simulink library "VISMODAL_MASTER"  (Simulink 8.6)
settings: Solver=VariableStepAuto  StartTime=0.0  StopTime=10.0  RelTol=1e-3
libraries: VIS_LIB x140, cdsFilt x34, cdsMuxMatrix x6, VISMODAL_MASTER x1
(part 2 of 5)

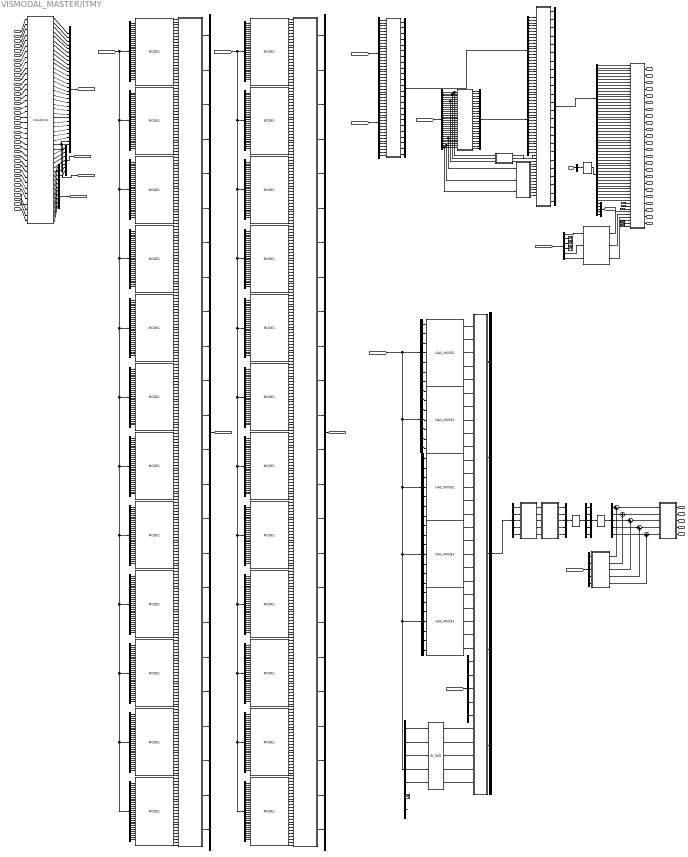
== system VISMODAL_MASTER/ITMY ==
  MCPS_V1 : Inport
  MCPS_V2 : Inport  Port=2
  MCPS_V3 : Inport  Port=3
  MCPS_H1 : Inport  Port=4
  MCPS_H2 : Inport  Port=5
  MCPS_H3 : Inport  Port=6
  IMPS_V1 : Inport  Port=7
  IMPS_V2 : Inport  Port=8
  IMPS_V3 : Inport  Port=9
  IMPS_H1 : Inport  Port=10
  IMPS_H2 : Inport  Port=11
  IMPS_H3 : Inport  Port=12
  TILT_SEG1 : Inport  Port=13
  TILT_SEG2 : Inport  Port=14
  TILT_SEG3 : Inport  Port=15
  TILT_SEG4 : Inport  Port=16
  LEN_SEG1 : Inport  Port=17
  LEN_SEG2 : Inport  Port=18
  LEN_SEG3 : Inport  Port=19
  LEN_SEG4 : Inport  Port=20
  BFLVDT_V1 : Inport  Port=21
  BFLVDT_V2 : Inport  Port=22
  BFLVDT_V3 : Inport  Port=23
  BFLVDT_H1 : Inport  Port=24
  BFLVDT_H2 : Inport  Port=25
  BFLVDT_H3 : Inport  Port=26
  IPLVDT_H1 : Inport  Port=27
  IPLVDT_H2 : Inport  Port=28
  IPLVDT_H3 : Inport  Port=29
  MNSEG1 : Inport  Port=30
  MNSEG2 : Inport  Port=31
  MNSEG3 : Inport  Port=32
  MNSEG4 : Inport  Port=33
  F0 : Inport  Port=34
  F1 : Inport  Port=35
  F2 : Inport  Port=36
  F3 : Inport  Port=37
  BF : Inport  Port=38
  QUAEXC : Inport  Port=39
  AI_GAS : Subsystem
  COILOUT_GAS : Subsystem
  DAMP : Subsystem
  DAMP_GAS : VISMODAL_MASTER/ITMY/AI_GAS
  DIAG : VIS_LIB/MODAL/inputproc
  DRIVEDECPL_GAS : cdsMuxMatrix/Subsystem  Tag=cdsMuxMatrix  Description=Any size matrix. Inputs and outputs must be connected using Mux and Demux parts.
      settings: AttributesFormatString=%<Tag>
  Demux{,2..24,27} (25 alike) : Demux  Outputs=30
  Demux{1,25..26,29,39} (5 alike) : Demux  Outputs=24
  Demux{28,30..33,41} (6 alike) : Demux  Outputs=7
  Demux{34..38} (5 alike) : Demux  Outputs=5
  Demux40 : Demux  Outputs=29
  Demux42 : Demux  Outputs=6
  EUL2COIL_GAS : cdsMuxMatrix/Subsystem  Tag=cdsMuxMatrix  Description=Any size matrix. Inputs and outputs must be connected using Mux and Demux parts.
      settings: AttributesFormatString=%<Tag>
  GASDC : Subsystem
  GAS_MODE{1..5} (5 alike) : VIS_LIB/MODAL/GAS_MODE1
  Ground{8..9,11,13,15,18} (6 alike) : Ground
  IPDC : Subsystem
  MNOL_SERVO_MN : Subsystem
  MODE{1..24} (24 alike) : VIS_LIB/MODAL/MODE1
  Mux : Mux  Inputs=30
  Mux{1..2,4..5,9} (5 alike) : Mux  Inputs=24
  Mux10 : Mux  Inputs=1
  Mux{6..8,11,13} (5 alike) : Mux  Inputs=5
  Mux12 : Mux  Inputs=6
  Mux3 : Mux  Inputs=7
  QUAEXC_SEL : cdsMuxMatrix/Subsystem  Tag=cdsMuxMatrix  Description=Any size matrix. Inputs and outputs must be connected using Mux and Demux parts.
      settings: AttributesFormatString=%<Tag>
  SUM_GAS : Subsystem
  Subsystem : Subsystem
  Sum{5..9} (5 alike) : Sum  Inputs=|++
  TMOL : Subsystem
  Terminator{,1..3} (4 alike) : Terminator
  sum : Subsystem
  sum1 : Subsystem
  sum10 : Subsystem
  sum2 : Subsystem
  sum3 : Subsystem
  IPLo : Outport
  IPTo : Outport  Port=2
  IPYo : Outport  Port=3
  BFLo : Outport  Port=4
  BFTo : Outport  Port=5
  BFVo : Outport  Port=6
  BFRo : Outport  Port=7
  BFPo : Outport  Port=8
  BFYo : Outport  Port=9
  MNLo : Outport  Port=10
  MNTo : Outport  Port=11
  MNVo : Outport  Port=12
  MNRo : Outport  Port=13
  MNPo : Outport  Port=14
  MNYo : Outport  Port=15
  IMLo : Outport  Port=16
  IMTo : Outport  Port=17
  IMVo : Outport  Port=18
  IMRo : Outport  Port=19
  IMPo : Outport  Port=20
  IMYo : Outport  Port=21
  TMLo : Outport  Port=22
  TMPo : Outport  Port=23
  TMYo : Outport  Port=24
  F0out : Outport  Port=25
  F1out : Outport  Port=26
  F2out : Outport  Port=27
  F3out : Outport  Port=28
  BFout : Outport  Port=29
  wires:
  Mux/1 -> [Signal]
  [Signal] -> Demux27/1
  DAMP/1(IPLo) -> Mux4/1
  DAMP/2(IPTo) -> Mux4/2
  DAMP/3(IPYo) -> Mux4/3
  DAMP/4(BFLo) -> Mux4/4
  DAMP/5(BFTo) -> Mux4/5
  DAMP/6(BFVo) -> Mux4/6
  DAMP/7(BFRo) -> Mux4/7
  DAMP/8(BFPo) -> Mux4/8
  DAMP/9(BFYo) -> Mux4/9
  DAMP/10(MNLo) -> Mux4/10
  DAMP/11(MNTo) -> Mux4/11
  DAMP/12(MNVo) -> Mux4/12
  DAMP/13(MNRo) -> Mux4/13
  DAMP/14(MNPo) -> Mux4/14
  DAMP/15(MNYo) -> Mux4/15
  DAMP/16(IMLo) -> Mux4/16
  DAMP/17(IMTo) -> Mux4/17
  DAMP/18(IMVo) -> Mux4/18
  DAMP/19(IMRo) -> Mux4/19
  DAMP/20(IMPo) -> Mux4/20
  DAMP/21(IMYo) -> Mux4/21
  DAMP/22(TMLo) -> Mux4/22
  DAMP/23(TMPo) -> Mux4/23
  DAMP/24(TMYo) -> Mux4/24
  Mux4/1 -> Demux29/1
  Demux29/1 -> sum10/25(IPL2)
  Demux29/2 -> sum10/26(IPT2)
  Demux29/3 -> sum10/27(IPY2)
  Demux29/4 -> sum10/28(BFL2)
  Demux29/5 -> sum10/29(BFT2)
  Demux29/6 -> sum10/30(BFV2)
  Demux29/7 -> sum10/31(BFR2)
  Demux29/8 -> sum10/32(BFP2)
  Demux29/9 -> sum10/33(BFY2)
  Demux29/10 -> sum10/34(MNL2)
  Demux29/11 -> sum10/35(MNT2)
  Demux29/12 -> sum10/36(MNV2)
  Demux29/13 -> sum10/37(MNR2)
  Demux29/14 -> sum10/38(MNP2)
  Demux29/15 -> sum10/39(MNY2)
  Demux29/16 -> sum10/40(IML2)
  Demux29/17 -> sum10/41(IMT2)
  Demux29/18 -> sum10/42(IMV2)
  Demux29/19 -> sum10/43(IMR2)
  Demux29/20 -> sum10/44(IMP2)
  Demux29/21 -> sum10/45(IMY2)
  Demux29/22 -> sum10/46(TML2)
  Demux29/23 -> sum10/47(TMP2)
  Demux29/24 -> sum10/48(TMY2)
  Demux27/1 -> IPDC/1(IPL), DAMP/1(IPL)
  Demux27/2 -> IPDC/2(IPT), DAMP/2(IPT)
  Demux27/3 -> DAMP/3(IPV)
  Demux27/4 -> DAMP/4(IPR)
  Demux27/5 -> DAMP/5(IPP)
  Demux27/6 -> IPDC/3(IPY), DAMP/6(IPY)
  Demux27/7 -> DAMP/7(BFL)
  Demux27/8 -> DAMP/8(BFT)
  Demux27/9 -> DAMP/9(BFV)
  Demux27/10 -> DAMP/10(BFR)
  Demux27/11 -> DAMP/11(BFP)
  Demux27/12 -> DAMP/12(BFY)
  Demux27/13 -> DAMP/13(MNL)
  Demux27/14 -> DAMP/14(MLT)
  Demux27/15 -> DAMP/15(MNV)
  Demux27/16 -> DAMP/16(MNR)
  Demux27/17 -> DAMP/17(MNP)
  Demux27/18 -> DAMP/18(MNY)
  Demux27/19 -> DAMP/19(IML)
  Demux27/20 -> DAMP/20(IMT)
  Demux27/21 -> DAMP/21(IMV)
  Demux27/22 -> DAMP/22(IMR)
  Demux27/23 -> DAMP/23(IMP)
  Demux27/24 -> DAMP/24(IMY)
  Demux27/26 -> DAMP/26(TMT)
  Demux27/27 -> DAMP/27(TMV)
  Demux27/28 -> DAMP/28(TMR)
  Demux27/29 -> TMOL/2(OLP), DAMP/29(TMP)
  Demux27/30 -> TMOL/3(OLY), DAMP/30(TMY)
  DIAG/1 -> Mux/1
  DIAG/2 -> Mux/2
  DIAG/3 -> Mux/3
  DIAG/4 -> Mux/4
  DIAG/5 -> Mux/5
  DIAG/6 -> Mux/6
  DIAG/7 -> Mux/7
  DIAG/8 -> Mux/8
  DIAG/9 -> Mux/9
  DIAG/10 -> Mux/10
  DIAG/11 -> Mux/11
  DIAG/12 -> Mux/12
  DIAG/13 -> Mux/13
  DIAG/14 -> Mux/14
  DIAG/15 -> Mux/15
  DIAG/16 -> Mux/16
  DIAG/17 -> Mux/17
  DIAG/18 -> Mux/18
  DIAG/19 -> Mux/19
  DIAG/20 -> Mux/20
  DIAG/21 -> Mux/21
  DIAG/22 -> Mux/22
  DIAG/23 -> Mux/23
  DIAG/24 -> Mux/24
  DIAG/25 -> Mux/25
  DIAG/26 -> Mux/26
  DIAG/27 -> Mux/27
  DIAG/28 -> Mux/28
  DIAG/29 -> Mux3/6, Mux/29
  DIAG/30 -> Mux3/7, Mux/30
  IPLVDT_H1/1 -> DIAG/1
  IPLVDT_H2/1 -> DIAG/2
  IPLVDT_H3/1 -> DIAG/3
  BFLVDT_V1/1 -> DIAG/4
  BFLVDT_V2/1 -> DIAG/5
  BFLVDT_V3/1 -> DIAG/6
  BFLVDT_H1/1 -> DIAG/7
  BFLVDT_H2/1 -> DIAG/8
  BFLVDT_H3/1 -> DIAG/9
  MCPS_V1/1 -> DIAG/10
  MCPS_V2/1 -> DIAG/11
  MCPS_V3/1 -> DIAG/12
  MCPS_H1/1 -> DIAG/13
  MCPS_H2/1 -> DIAG/14
  MCPS_H3/1 -> DIAG/15
  IMPS_V1/1 -> DIAG/16
  IMPS_V2/1 -> DIAG/17
  IMPS_V3/1 -> DIAG/18
  IMPS_H1/1 -> DIAG/19
  IMPS_H2/1 -> DIAG/20
  IMPS_H3/1 -> DIAG/21
  TILT_SEG1/1 -> DIAG/22
  TILT_SEG2/1 -> DIAG/23
  TILT_SEG3/1 -> DIAG/24
  TILT_SEG4/1 -> DIAG/25
  LEN_SEG1/1 -> DIAG/26
  LEN_SEG2/1 -> DIAG/27
  LEN_SEG3/1 -> DIAG/28
  LEN_SEG4/1 -> DIAG/29
  MNSEG2/1 -> DIAG/31
  MNSEG1/1 -> DIAG/30
  MNSEG3/1 -> DIAG/32
  MNSEG4/1 -> DIAG/33
  sum/1(IPL) -> Mux1/1
  sum/2(IPT) -> Mux1/2
  sum/3(IPY) -> Mux1/3
  sum/4(BFL) -> Mux1/4
  sum/5(BFT) -> Mux1/5
  sum/6(BFV) -> Mux1/6
  sum/7(BFR) -> Mux1/7
  sum/8(BFP) -> Mux1/8
  sum/9(BFY) -> Mux1/9
  sum/10(MNL) -> Mux1/10
  sum/11(MNT) -> Mux1/11
  sum/12(MNV) -> Mux1/12
  sum/13(MNR) -> Mux1/13
  sum/14(MNP) -> Mux1/14
  sum/15(MNY) -> Mux1/15
  sum/16(IML) -> Mux1/16
  sum/17(IMT) -> Mux1/17
  sum/18(IMV) -> Mux1/18
  sum/19(IMR) -> Mux1/19
  sum/20(IMP) -> Mux1/20
  sum/21(IMY) -> Mux1/21
  sum/22(TML) -> Mux1/22
  sum/23(TMP) -> Mux1/23
  sum/24(TMY) -> Mux1/24
  MODE1/1 -> sum/1(IPL1)
  MODE1/2 -> sum/2(IPT1)
  MODE1/3 -> sum/3(IPY1)
  MODE1/4 -> sum/4(BFL1)
  MODE1/5 -> sum/5(BFT1)
  MODE1/6 -> sum/6(BFV1)
  MODE1/7 -> sum/7(BFR1)
  MODE1/8 -> sum/8(BFP1)
  MODE1/9 -> sum/9(BFY1)
  MODE1/10 -> sum/10(MNL1)
  MODE1/11 -> sum/11(MNT1)
  MODE1/12 -> sum/12(MNV1)
  MODE1/13 -> sum/13(MNR1)
  MODE1/14 -> sum/14(MNP1)
  MODE1/15 -> sum/15(MNY1)
  MODE1/16 -> sum/16(IML1)
  MODE1/17 -> sum/17(IMT1)
  MODE1/18 -> sum/18(IMV1)
  MODE1/19 -> sum/19(IMR1)
  MODE1/20 -> sum/20(IMP1)
  MODE1/21 -> sum/21(IMY1)
  MODE1/22 -> sum/22(TML1)
  MODE1/23 -> sum/23(TMP1)
  MODE1/24 -> sum/24(TMY1)
  Demux/1 -> MODE1/1
  Demux/2 -> MODE1/2
  Demux/3 -> MODE1/3
  Demux/4 -> MODE1/4
  Demux/5 -> MODE1/5
  Demux/6 -> MODE1/6
  Demux/7 -> MODE1/7
  Demux/8 -> MODE1/8
  Demux/9 -> MODE1/9
  Demux/10 -> MODE1/10
  Demux/11 -> MODE1/11
  Demux/12 -> MODE1/12
  Demux/13 -> MODE1/13
  Demux/14 -> MODE1/14
  Demux/15 -> MODE1/15
  Demux/16 -> MODE1/16
  Demux/17 -> MODE1/17
  Demux/18 -> MODE1/18
  Demux/19 -> MODE1/19
  Demux/20 -> MODE1/20
  Demux/21 -> MODE1/21
  Demux/22 -> MODE1/22
  Demux/23 -> MODE1/23
  Demux/24 -> MODE1/24
  Demux/25 -> MODE1/25
  Demux/26 -> MODE1/26
  Demux/27 -> MODE1/27
  Demux/28 -> MODE1/28
  Demux/29 -> MODE1/29
  Demux/30 -> MODE1/30
  Demux2/1 -> MODE2/1
  Demux2/2 -> MODE2/2
  Demux2/3 -> MODE2/3
  Demux2/4 -> MODE2/4
  Demux2/5 -> MODE2/5
  Demux2/6 -> MODE2/6
  Demux2/7 -> MODE2/7
  Demux2/8 -> MODE2/8
  Demux2/9 -> MODE2/9
  Demux2/10 -> MODE2/10
  Demux2/11 -> MODE2/11
  Demux2/12 -> MODE2/12
  Demux2/13 -> MODE2/13
  Demux2/14 -> MODE2/14
  Demux2/15 -> MODE2/15
  Demux2/16 -> MODE2/16
  Demux2/17 -> MODE2/17
  Demux2/18 -> MODE2/18
  Demux2/19 -> MODE2/19
  Demux2/20 -> MODE2/20
  Demux2/21 -> MODE2/21
  Demux2/22 -> MODE2/22
  Demux2/23 -> MODE2/23
  Demux2/24 -> MODE2/24
  Demux2/25 -> MODE2/25
  Demux2/26 -> MODE2/26
  MODE2/1 -> sum/25(IPL2)
  MODE2/2 -> sum/26(IPT2)
  MODE2/3 -> sum/27(IPY2)
  MODE2/4 -> sum/28(BFL2)
  MODE2/5 -> sum/29(BFT2)
  MODE2/6 -> sum/30(BFV2)
  MODE2/7 -> sum/31(BFR2)
  MODE2/8 -> sum/32(BFP2)
  MODE2/9 -> sum/33(BFY2)
  MODE2/10 -> sum/34(MNL2)
  MODE2/11 -> sum/35(MNT2)
  MODE2/12 -> sum/36(MNV2)
  MODE2/13 -> sum/37(MNR2)
  MODE2/14 -> sum/38(MNP2)
  MODE2/15 -> sum/39(MNY2)
  MODE2/16 -> sum/40(IML2)
  MODE2/17 -> sum/41(IMT2)
  MODE2/18 -> sum/42(IMV2)
  MODE2/19 -> sum/43(IMR2)
  MODE2/20 -> sum/44(IMP2)
  MODE2/21 -> sum/45(IMY2)
  MODE2/22 -> sum/46(TML2)
  MODE2/23 -> sum/47(TMP2)
  MODE2/24 -> sum/48(TMY2)
  Demux2/27 -> MODE2/27
  Demux2/28 -> MODE2/28
  Demux2/29 -> MODE2/29
  Demux2/30 -> MODE2/30
  Demux3/1 -> MODE3/1
  Demux3/2 -> MODE3/2
  Demux3/3 -> MODE3/3
  Demux3/4 -> MODE3/4
  Demux3/5 -> MODE3/5
  Demux3/6 -> MODE3/6
  Demux3/7 -> MODE3/7
  Demux3/8 -> MODE3/8
  Demux3/9 -> MODE3/9
  Demux3/10 -> MODE3/10
  Demux3/11 -> MODE3/11
  Demux3/12 -> MODE3/12
  Demux3/13 -> MODE3/13
  Demux3/14 -> MODE3/14
  Demux3/15 -> MODE3/15
  Demux3/16 -> MODE3/16
  Demux3/17 -> MODE3/17
  Demux3/18 -> MODE3/18
  Demux3/19 -> MODE3/19
  Demux3/20 -> MODE3/20
  Demux3/21 -> MODE3/21
  Demux3/22 -> MODE3/22
  Demux3/23 -> MODE3/23
  Demux3/24 -> MODE3/24
  Demux3/25 -> MODE3/25
  Demux3/26 -> MODE3/26
  MODE3/1 -> sum/49(IPL3)
  MODE3/2 -> sum/50(IPT3)
  MODE3/3 -> sum/51(IPY3)
  MODE3/4 -> sum/52(BFL3)
  MODE3/5 -> sum/53(BFT3)
  MODE3/6 -> sum/54(BFV3)
  MODE3/7 -> sum/55(BFR3)
  MODE3/8 -> sum/56(BFP3)
  MODE3/9 -> sum/57(BFY3)
  MODE3/10 -> sum/58(MNL3)
  MODE3/11 -> sum/59(MNT3)
  MODE3/12 -> sum/60(MNV3)
  MODE3/13 -> sum/61(MNR3)
  MODE3/14 -> sum/62(MNP3)
  MODE3/15 -> sum/63(MNY3)
  MODE3/16 -> sum/64(IML3)
  MODE3/17 -> sum/65(IMT3)
  MODE3/18 -> sum/66(IMV3)
  MODE3/19 -> sum/67(IMR3)
  MODE3/20 -> sum/68(IMP3)
  MODE3/21 -> sum/69(IMY3)
  MODE3/22 -> sum/70(TML3)
  MODE3/23 -> sum/71(TMP3)
  MODE3/24 -> sum/72(TMY3)
  Demux3/27 -> MODE3/27
  Demux3/28 -> MODE3/28
  Demux3/29 -> MODE3/29
  Demux3/30 -> MODE3/30
  Demux4/1 -> MODE4/1
  Demux4/2 -> MODE4/2
  Demux4/3 -> MODE4/3
  Demux4/4 -> MODE4/4
  Demux4/5 -> MODE4/5
  Demux4/6 -> MODE4/6
  Demux4/7 -> MODE4/7
  Demux4/8 -> MODE4/8
  Demux4/9 -> MODE4/9
  Demux4/10 -> MODE4/10
  Demux4/11 -> MODE4/11
  Demux4/12 -> MODE4/12
  Demux4/13 -> MODE4/13
  Demux4/14 -> MODE4/14
  Demux4/15 -> MODE4/15
  Demux4/16 -> MODE4/16
  Demux4/17 -> MODE4/17
  Demux4/18 -> MODE4/18
  Demux4/19 -> MODE4/19
  Demux4/20 -> MODE4/20
  Demux4/21 -> MODE4/21
  Demux4/22 -> MODE4/22
  Demux4/23 -> MODE4/23
  Demux4/24 -> MODE4/24
  Demux4/25 -> MODE4/25
  Demux4/26 -> MODE4/26
  MODE4/1 -> sum/73(IPL4)
  MODE4/2 -> sum/74(IPT4)
  MODE4/3 -> sum/75(IPY4)
  MODE4/4 -> sum/76(BFL4)
  MODE4/5 -> sum/77(BFT4)
  MODE4/6 -> sum/78(BFV4)
  MODE4/7 -> sum/79(BFR4)
  MODE4/8 -> sum/80(BFP4)
  MODE4/9 -> sum/81(BFY4)
  MODE4/10 -> sum/82(MNL4)
  MODE4/11 -> sum/83(MNT4)
  MODE4/12 -> sum/84(MNV4)
  MODE4/13 -> sum/85(MNR4)
  MODE4/14 -> sum/86(MNP4)
  MODE4/15 -> sum/87(MNY4)
  MODE4/16 -> sum/88(IML4)
  MODE4/17 -> sum/89(IMT4)
  MODE4/18 -> sum/90(IMV4)
  MODE4/19 -> sum/91(IMR4)
  MODE4/20 -> sum/92(IMP4)
  MODE4/21 -> sum/93(IMY4)
  MODE4/22 -> sum/94(TML4)
  MODE4/23 -> sum/95(TMP4)
  MODE4/24 -> sum/96(TMY4)
  Demux4/27 -> MODE4/27
  Demux4/28 -> MODE4/28
  Demux4/29 -> MODE4/29
  Demux4/30 -> MODE4/30
  MODE5/1 -> sum/97(IPL5)
  MODE5/2 -> sum/98(IPT5)
  MODE5/3 -> sum/99(IPY5)
  MODE5/4 -> sum/100(BFL5)
  MODE5/5 -> sum/101(BFT5)
  MODE5/6 -> sum/102(BFV5)
  MODE5/7 -> sum/103(BFR5)
  MODE5/8 -> sum/104(BFP5)
  MODE5/9 -> sum/105(BFY5)
  MODE5/10 -> sum/106(MNL5)
  MODE5/11 -> sum/107(MNT5)
  MODE5/12 -> sum/108(MNV5)
  MODE5/13 -> sum/109(MNR5)
  MODE5/14 -> sum/110(MNP5)
  MODE5/15 -> sum/111(MNY5)
  MODE5/16 -> sum/112(IML5)
  MODE5/17 -> sum/113(IMT5)
  MODE5/18 -> sum/114(IMV5)
  MODE5/19 -> sum/115(IMR5)
  MODE5/20 -> sum/116(IMP5)
  MODE5/21 -> sum/117(IMY5)
  MODE5/22 -> sum/118(TML5)
  MODE5/23 -> sum/119(TMP5)
  MODE5/24 -> sum/120(TMY5)
  Demux5/1 -> MODE5/1
  Demux5/2 -> MODE5/2
  Demux5/3 -> MODE5/3
  Demux5/4 -> MODE5/4
  Demux5/5 -> MODE5/5
  Demux5/6 -> MODE5/6
  Demux5/7 -> MODE5/7
  Demux5/8 -> MODE5/8
  Demux5/9 -> MODE5/9
  Demux5/10 -> MODE5/10
  Demux5/11 -> MODE5/11
  Demux5/12 -> MODE5/12
  Demux5/13 -> MODE5/13
  Demux5/14 -> MODE5/14
  Demux5/15 -> MODE5/15
  Demux5/16 -> MODE5/16
  Demux5/17 -> MODE5/17
  Demux5/18 -> MODE5/18
  Demux5/19 -> MODE5/19
  Demux5/20 -> MODE5/20
  Demux5/21 -> MODE5/21
  Demux5/22 -> MODE5/22
  Demux5/23 -> MODE5/23
  Demux5/24 -> MODE5/24
  Demux5/25 -> MODE5/25
  Demux5/26 -> MODE5/26
  Demux5/27 -> MODE5/27
  Demux5/28 -> MODE5/28
  Demux5/29 -> MODE5/29
  Demux5/30 -> MODE5/30
  Demux6/1 -> MODE6/1
  Demux6/2 -> MODE6/2
  Demux6/3 -> MODE6/3
  Demux6/4 -> MODE6/4
  Demux6/5 -> MODE6/5
  Demux6/6 -> MODE6/6
  Demux6/7 -> MODE6/7
  Demux6/8 -> MODE6/8
  Demux6/9 -> MODE6/9
  Demux6/10 -> MODE6/10
  Demux6/11 -> MODE6/11
  Demux6/12 -> MODE6/12
  Demux6/13 -> MODE6/13
  Demux6/14 -> MODE6/14
  Demux6/15 -> MODE6/15
  Demux6/16 -> MODE6/16
  Demux6/17 -> MODE6/17
  Demux6/18 -> MODE6/18
  Demux6/19 -> MODE6/19
  Demux6/20 -> MODE6/20
  Demux6/21 -> MODE6/21
  Demux6/22 -> MODE6/22
  Demux6/23 -> MODE6/23
  Demux6/24 -> MODE6/24
  Demux6/25 -> MODE6/25
  Demux6/26 -> MODE6/26
  MODE6/1 -> sum/121(IPL6)
  MODE6/2 -> sum/122(IPT6)
  MODE6/3 -> sum/123(IPY6)
  MODE6/4 -> sum/124(BFL6)
  MODE6/5 -> sum/125(BFT6)
  MODE6/6 -> sum/126(BFV6)
  MODE6/7 -> sum/127(BFR6)
  MODE6/8 -> sum/128(BFP6)
  MODE6/9 -> sum/129(BFY6)
  MODE6/10 -> sum/130(MNL6)
  MODE6/11 -> sum/131(MNT6)
  MODE6/12 -> sum/132(MNV6)
  MODE6/13 -> sum/133(MNR6)
  MODE6/14 -> sum/134(MNP6)
  MODE6/15 -> sum/135(MNY6)
  MODE6/16 -> sum/136(IML6)
  MODE6/17 -> sum/137(IMT6)
  MODE6/18 -> sum/138(IMV6)
  MODE6/19 -> sum/139(IMR6)
  MODE6/20 -> sum/140(IMP6)
  MODE6/21 -> sum/141(IMY6)
  MODE6/22 -> sum/142(TML6)
  MODE6/23 -> sum/143(TMP6)
  MODE6/24 -> sum/144(TMY6)
  Demux6/27 -> MODE6/27
  Demux6/28 -> MODE6/28
  Demux6/29 -> MODE6/29
  Demux6/30 -> MODE6/30
  Demux7/1 -> MODE7/1
  Demux7/2 -> MODE7/2
  Demux7/3 -> MODE7/3
  Demux7/4 -> MODE7/4
  Demux7/5 -> MODE7/5
  Demux7/6 -> MODE7/6
  Demux7/7 -> MODE7/7
  Demux7/8 -> MODE7/8
  Demux7/9 -> MODE7/9
  Demux7/10 -> MODE7/10
  Demux7/11 -> MODE7/11
  Demux7/12 -> MODE7/12
  Demux7/13 -> MODE7/13
  Demux7/14 -> MODE7/14
  Demux7/15 -> MODE7/15
  Demux7/16 -> MODE7/16
  Demux7/17 -> MODE7/17
  Demux7/18 -> MODE7/18
  Demux7/19 -> MODE7/19
  Demux7/20 -> MODE7/20
  Demux7/21 -> MODE7/21
  Demux7/22 -> MODE7/22
  Demux7/23 -> MODE7/23
  Demux7/24 -> MODE7/24
  Demux7/25 -> MODE7/25
  Demux7/26 -> MODE7/26
  MODE7/1 -> sum/145(IPL7)
  MODE7/2 -> sum/146(IPT7)
  MODE7/3 -> sum/147(IPY7)
  MODE7/4 -> sum/148(BFL7)
  MODE7/5 -> sum/149(BFT7)
  MODE7/6 -> sum/150(BFV7)
  MODE7/7 -> sum/151(BFR7)
  MODE7/8 -> sum/152(BFP7)
  MODE7/9 -> sum/153(BFY7)
  MODE7/10 -> sum/154(MNL7)
  MODE7/11 -> sum/155(MNT7)
  MODE7/12 -> sum/156(MNV7)
  MODE7/13 -> sum/157(MNR7)
  MODE7/14 -> sum/158(MNP7)
  MODE7/15 -> sum/159(MNY7)
  MODE7/16 -> sum/160(IML7)
  MODE7/17 -> sum/161(IMT7)
  MODE7/18 -> sum/162(IMV7)
  MODE7/19 -> sum/163(IMR7)
  MODE7/20 -> sum/164(IMP7)
  MODE7/21 -> sum/165(IMY7)
  MODE7/22 -> sum/166(TML7)
  MODE7/23 -> sum/167(TMP7)
  MODE7/24 -> sum/168(TMY7)
  Demux7/27 -> MODE7/27
  Demux7/28 -> MODE7/28
  Demux7/29 -> MODE7/29
  Demux7/30 -> MODE7/30
  Demux8/1 -> MODE8/1
  Demux8/2 -> MODE8/2
  Demux8/3 -> MODE8/3
  Demux8/4 -> MODE8/4
  Demux8/5 -> MODE8/5
  Demux8/6 -> MODE8/6
  Demux8/7 -> MODE8/7
  Demux8/8 -> MODE8/8
  Demux8/9 -> MODE8/9
  Demux8/10 -> MODE8/10
  Demux8/11 -> MODE8/11
  Demux8/12 -> MODE8/12
  Demux8/13 -> MODE8/13
  Demux8/14 -> MODE8/14
  Demux8/15 -> MODE8/15
  Demux8/16 -> MODE8/16
  Demux8/17 -> MODE8/17
  Demux8/18 -> MODE8/18
  Demux8/19 -> MODE8/19
  Demux8/20 -> MODE8/20
  Demux8/21 -> MODE8/21
  Demux8/22 -> MODE8/22
  Demux8/23 -> MODE8/23
  Demux8/24 -> MODE8/24
  Demux8/25 -> MODE8/25
  Demux8/26 -> MODE8/26
  MODE8/1 -> sum/169(IPL8)
  MODE8/2 -> sum/170(IPT8)
  MODE8/3 -> sum/171(IPY8)
  MODE8/4 -> sum/172(BFL8)
  MODE8/5 -> sum/173(BFT8)
  MODE8/6 -> sum/174(BFV8)
  MODE8/7 -> sum/175(BFR8)
  MODE8/8 -> sum/176(BFP8)
  MODE8/9 -> sum/177(BFY8)
  MODE8/10 -> sum/178(MNL8)
  MODE8/11 -> sum/179(MNT8)
  MODE8/12 -> sum/180(MNV8)
  MODE8/13 -> sum/181(MNR8)
  MODE8/14 -> sum/182(MNP8)
  MODE8/15 -> sum/183(MNY8)
  MODE8/16 -> sum/184(IML8)
  MODE8/17 -> sum/185(IMT8)
  MODE8/18 -> sum/186(IMV8)
  MODE8/19 -> sum/187(IMR8)
  MODE8/20 -> sum/188(IMP8)
  MODE8/21 -> sum/189(IMY8)
  MODE8/22 -> sum/190(TML8)
  MODE8/23 -> sum/191(TMP8)
  MODE8/24 -> sum/192(TMY8)
  Demux8/27 -> MODE8/27
  Demux8/28 -> MODE8/28
  Demux8/29 -> MODE8/29
  Demux8/30 -> MODE8/30
  MODE9/10 -> sum/202(MNL9)
  MODE9/11 -> sum/203(MNT9)
  MODE9/12 -> sum/204(MNV9)
  MODE9/13 -> sum/205(MNR9)
  MODE9/14 -> sum/206(MNP9)
  MODE9/15 -> sum/207(MNY9)
  MODE9/16 -> sum/208(IML9)
  MODE9/17 -> sum/209(IMT9)
  MODE9/18 -> sum/210(IMV9)
  MODE9/19 -> sum/211(IMR9)
  MODE9/20 -> sum/212(IMP9)
  MODE9/21 -> sum/213(IMY9)
  MODE9/22 -> sum/214(TML9)
  MODE9/23 -> sum/215(TMP9)
  MODE9/24 -> sum/216(TMY9)
  Demux9/11 -> MODE9/11
  Demux9/12 -> MODE9/12
  Demux9/13 -> MODE9/13
  Demux9/14 -> MODE9/14
  Demux9/15 -> MODE9/15
  Demux9/16 -> MODE9/16
  Demux9/17 -> MODE9/17
  Demux9/18 -> MODE9/18
  Demux9/19 -> MODE9/19
  Demux9/20 -> MODE9/20
  Demux9/21 -> MODE9/21
  Demux9/22 -> MODE9/22
  Demux9/23 -> MODE9/23
  Demux9/24 -> MODE9/24
  Demux9/25 -> MODE9/25
  Demux9/26 -> MODE9/26
  Demux9/27 -> MODE9/27
  Demux9/28 -> MODE9/28
  Demux9/29 -> MODE9/29
  Demux9/30 -> MODE9/30
  Demux10/1 -> MODE10/1
  Demux10/2 -> MODE10/2
  Demux10/3 -> MODE10/3
  Demux10/4 -> MODE10/4
  Demux10/5 -> MODE10/5
  Demux10/6 -> MODE10/6
  Demux10/7 -> MODE10/7
  Demux10/8 -> MODE10/8
  Demux10/9 -> MODE10/9
  Demux10/10 -> MODE10/10
  Demux10/11 -> MODE10/11
  Demux10/12 -> MODE10/12
  Demux10/13 -> MODE10/13
  Demux10/14 -> MODE10/14
  Demux10/15 -> MODE10/15
  Demux10/16 -> MODE10/16
  Demux10/17 -> MODE10/17
  Demux10/18 -> MODE10/18
  Demux10/19 -> MODE10/19
  Demux10/20 -> MODE10/20
  Demux10/21 -> MODE10/21
  Demux10/22 -> MODE10/22
  Demux10/23 -> MODE10/23
  Demux10/24 -> MODE10/24
  Demux10/25 -> MODE10/25
  Demux10/26 -> MODE10/26
  MODE10/1 -> sum/217(IPL10)
  MODE10/2 -> sum/218(IPT10)
  MODE10/3 -> sum/219(IPY10)
  MODE10/4 -> sum/220(BFL10)
  MODE10/5 -> sum/221(BFT10)
  MODE10/6 -> sum/222(BFV10)
  MODE10/7 -> sum/223(BFR10)
  MODE10/8 -> sum/224(BFP10)
  MODE10/9 -> sum/225(BFY10)
  MODE10/10 -> sum/226(MNL10)
  MODE10/11 -> sum/227(MNT10)
  MODE10/12 -> sum/228(MNV10)
  MODE10/13 -> sum/229(MNR10)
  MODE10/14 -> sum/230(MNP10)
  MODE10/15 -> sum/231(MNY10)
  MODE10/16 -> sum/232(IML10)
  MODE10/17 -> sum/233(IMT10)
  MODE10/18 -> sum/234(IMV10)
  MODE10/19 -> sum/235(IMR10)
  MODE10/20 -> sum/236(IMP10)
  MODE10/21 -> sum/237(IMY10)
  MODE10/22 -> sum/238(TML10)
  MODE10/23 -> sum/239(TMP10)
  MODE10/24 -> sum/240(TMY10)
  Demux10/27 -> MODE10/27
  Demux10/28 -> MODE10/28
  Demux10/29 -> MODE10/29
  Demux10/30 -> MODE10/30
  Demux11/1 -> MODE11/1
  Demux11/2 -> MODE11/2
  Demux11/3 -> MODE11/3
  Demux11/4 -> MODE11/4
  Demux11/5 -> MODE11/5
  Demux11/6 -> MODE11/6
  Demux11/7 -> MODE11/7
  Demux11/8 -> MODE11/8
  Demux11/9 -> MODE11/9
  Demux11/10 -> MODE11/10
  Demux11/11 -> MODE11/11
  Demux11/12 -> MODE11/12
  Demux11/13 -> MODE11/13
  Demux11/14 -> MODE11/14
  Demux11/15 -> MODE11/15
  Demux11/16 -> MODE11/16
  Demux11/17 -> MODE11/17
  Demux11/18 -> MODE11/18
  Demux11/19 -> MODE11/19
  Demux11/20 -> MODE11/20
  Demux11/21 -> MODE11/21
  Demux11/22 -> MODE11/22
  Demux11/23 -> MODE11/23
  Demux11/24 -> MODE11/24
  Demux11/25 -> MODE11/25
  Demux11/26 -> MODE11/26
  MODE11/1 -> sum/241(IPL11)
  MODE11/2 -> sum/242(IPT11)
  MODE11/3 -> sum/243(IPY11)
  MODE11/4 -> sum/244(BFL11)
  MODE11/5 -> sum/245(BFT11)
  MODE11/6 -> sum/246(BFV11)
  MODE11/7 -> sum/247(BFR11)
  MODE11/8 -> sum/248(BFP11)
  MODE11/9 -> sum/249(BFY11)
  MODE11/10 -> sum/250(MNL11)
  MODE11/11 -> sum/251(MNT11)
  MODE11/12 -> sum/252(MNV11)
  MODE11/13 -> sum/253(MNR11)
  MODE11/14 -> sum/254(MNP11)
  MODE11/15 -> sum/255(MNY11)
  MODE11/16 -> sum/256(IML11)
  MODE11/17 -> sum/257(IMT11)
  MODE11/18 -> sum/258(IMV11)
  MODE11/19 -> sum/259(IMR11)
  MODE11/20 -> sum/260(IMP11)
  MODE11/21 -> sum/261(IMY11)
  MODE11/22 -> sum/262(TML11)
  MODE11/23 -> sum/263(TMP11)
  MODE11/24 -> sum/264(TMY11)
  Demux11/27 -> MODE11/27
  Demux11/28 -> MODE11/28
  Demux11/29 -> MODE11/29
  Demux11/30 -> MODE11/30
  Demux12/1 -> MODE12/1
  Demux12/2 -> MODE12/2
  Demux12/3 -> MODE12/3
  Demux12/4 -> MODE12/4
  Demux12/5 -> MODE12/5
  Demux12/6 -> MODE12/6
  Demux12/7 -> MODE12/7
  Demux12/8 -> MODE12/8
  Demux12/9 -> MODE12/9
  Demux12/10 -> MODE12/10
  Demux12/11 -> MODE12/11
  Demux12/12 -> MODE12/12
  Demux12/13 -> MODE12/13
  Demux12/14 -> MODE12/14
  Demux12/15 -> MODE12/15
  Demux12/16 -> MODE12/16
  Demux12/17 -> MODE12/17
  Demux12/18 -> MODE12/18
  Demux12/19 -> MODE12/19
  Demux12/20 -> MODE12/20
  Demux12/21 -> MODE12/21
  Demux12/22 -> MODE12/22
  Demux12/23 -> MODE12/23
  Demux12/24 -> MODE12/24
  Demux12/25 -> MODE12/25
  Demux12/26 -> MODE12/26
  MODE12/1 -> sum/265(IPL12)
  MODE12/2 -> sum/266(IPT12)
  MODE12/3 -> sum/267(IPY12)
  MODE12/4 -> sum/268(BFL12)
  MODE12/5 -> sum/269(BFT12)
  MODE12/6 -> sum/270(BFV12)
  MODE12/7 -> sum/271(BFR12)
  MODE12/8 -> sum/272(BFP12)
  MODE12/9 -> sum/273(BFY12)
  MODE12/10 -> sum/274(MNL12)
  MODE12/11 -> sum/275(MNT12)
  MODE12/12 -> sum/276(MNV12)
  MODE12/13 -> sum/277(MNR12)
  MODE12/14 -> sum/278(MNP12)
  MODE12/15 -> sum/279(MNY12)
  MODE12/16 -> sum/280(IML12)
  MODE12/17 -> sum/281(IMT12)
  MODE12/18 -> sum/282(IMV12)
  MODE12/19 -> sum/283(IMR12)
  MODE12/20 -> sum/284(IMP12)
  MODE12/21 -> sum/285(IMY12)
  MODE12/22 -> sum/286(TML12)
  MODE12/23 -> sum/287(TMP12)
  MODE12/24 -> sum/288(TMY12)
  Demux12/27 -> MODE12/27
  Demux12/28 -> MODE12/28
  Demux12/29 -> MODE12/29
  Demux12/30 -> MODE12/30
  MODE9/1 -> sum/193(IPL9)
  MODE9/2 -> sum/194(IPT9)
  MODE9/3 -> sum/195(IPY9)
  MODE9/4 -> sum/196(BFL9)
  MODE9/5 -> sum/197(BFT9)
  MODE9/6 -> sum/198(BFV9)
  MODE9/7 -> sum/199(BFR9)
  MODE9/8 -> sum/200(BFP9)
  MODE9/9 -> sum/201(BFY9)
  Demux9/1 -> MODE9/1
  Demux9/2 -> MODE9/2
  Demux9/3 -> MODE9/3
  Demux9/4 -> MODE9/4
  Demux9/5 -> MODE9/5
  Demux9/6 -> MODE9/6
  Demux9/7 -> MODE9/7
  Demux9/8 -> MODE9/8
  Demux9/9 -> MODE9/9
  Demux9/10 -> MODE9/10
  sum1/1(IPL) -> Mux2/1
  sum1/2(IPT) -> Mux2/2
  sum1/3(IPY) -> Mux2/3
  sum1/4(BFL) -> Mux2/4
  sum1/5(BFT) -> Mux2/5
  sum1/6(BFV) -> Mux2/6
  sum1/7(BFR) -> Mux2/7
  sum1/8(BFP) -> Mux2/8
  sum1/9(BFY) -> Mux2/9
  sum1/10(MNL) -> Mux2/10
  sum1/11(MNT) -> Mux2/11
  sum1/12(MNV) -> Mux2/12
  sum1/13(MNR) -> Mux2/13
  sum1/14(MNP) -> Mux2/14
  sum1/15(MNY) -> Mux2/15
  sum1/16(IML) -> Mux2/16
  sum1/17(IMT) -> Mux2/17
  sum1/18(IMV) -> Mux2/18
  sum1/19(IMR) -> Mux2/19
  sum1/20(IMP) -> Mux2/20
  sum1/21(IMY) -> Mux2/21
  sum1/22(TML) -> Mux2/22
  sum1/23(TMP) -> Mux2/23
  sum1/24(TMY) -> Mux2/24
  MODE13/1 -> sum1/1(IPL1)
  MODE13/2 -> sum1/2(IPT1)
  MODE13/3 -> sum1/3(IPY1)
  MODE13/4 -> sum1/4(BFL1)
  MODE13/5 -> sum1/5(BFT1)
  MODE13/6 -> sum1/6(BFV1)
  MODE13/7 -> sum1/7(BFR1)
  MODE13/8 -> sum1/8(BFP1)
  MODE13/9 -> sum1/9(BFY1)
  MODE13/10 -> sum1/10(MNL1)
  MODE13/11 -> sum1/11(MNT1)
  MODE13/12 -> sum1/12(MNV1)
  MODE13/13 -> sum1/13(MNR1)
  MODE13/14 -> sum1/14(MNP1)
  MODE13/15 -> sum1/15(MNY1)
  MODE13/16 -> sum1/16(IML1)
  MODE13/17 -> sum1/17(IMT1)
  MODE13/18 -> sum1/18(IMV1)
  MODE13/19 -> sum1/19(IMR1)
  MODE13/20 -> sum1/20(IMP1)
  MODE13/21 -> sum1/21(IMY1)
  MODE13/22 -> sum1/22(TML1)
  MODE13/23 -> sum1/23(TMP1)
  MODE13/24 -> sum1/24(TMY1)
  Demux13/1 -> MODE13/1
  Demux13/2 -> MODE13/2
  Demux13/3 -> MODE13/3
  Demux13/4 -> MODE13/4
  Demux13/5 -> MODE13/5
  Demux13/6 -> MODE13/6
  Demux13/7 -> MODE13/7
  Demux13/8 -> MODE13/8
  Demux13/9 -> MODE13/9
  Demux13/10 -> MODE13/10
  Demux13/11 -> MODE13/11
  Demux13/12 -> MODE13/12
  Demux13/13 -> MODE13/13
  Demux13/14 -> MODE13/14
  Demux13/15 -> MODE13/15
  Demux13/16 -> MODE13/16
  Demux13/17 -> MODE13/17
  Demux13/18 -> MODE13/18
  Demux13/19 -> MODE13/19
  Demux13/20 -> MODE13/20
  Demux13/21 -> MODE13/21
  Demux13/22 -> MODE13/22
  Demux13/23 -> MODE13/23
  Demux13/24 -> MODE13/24
  Demux13/25 -> MODE13/25
  Demux13/26 -> MODE13/26
  Demux13/27 -> MODE13/27
  Demux13/28 -> MODE13/28
  Demux13/29 -> MODE13/29
  Demux13/30 -> MODE13/30
  Demux17/1 -> MODE17/1
  Demux17/2 -> MODE17/2
  Demux17/3 -> MODE17/3
  Demux17/4 -> MODE17/4
  Demux17/5 -> MODE17/5
  Demux17/6 -> MODE17/6
  Demux17/7 -> MODE17/7
  Demux17/8 -> MODE17/8
  Demux17/9 -> MODE17/9
  Demux17/10 -> MODE17/10
  Demux17/11 -> MODE17/11
  Demux17/12 -> MODE17/12
  Demux17/13 -> MODE17/13
  Demux17/14 -> MODE17/14
  Demux17/15 -> MODE17/15
  Demux17/16 -> MODE17/16
  Demux17/17 -> MODE17/17
  Demux17/18 -> MODE17/18
  Demux17/19 -> MODE17/19
  Demux17/20 -> MODE17/20
  Demux17/21 -> MODE17/21
  Demux17/22 -> MODE17/22
  Demux17/23 -> MODE17/23
  Demux17/24 -> MODE17/24
  Demux17/25 -> MODE17/25
  Demux17/26 -> MODE17/26
  MODE17/1 -> sum1/25(IPL2)
  MODE17/2 -> sum1/26(IPT2)
  MODE17/3 -> sum1/27(IPY2)
  MODE17/4 -> sum1/28(BFL2)
  MODE17/5 -> sum1/29(BFT2)
  MODE17/6 -> sum1/30(BFV2)
  MODE17/7 -> sum1/31(BFR2)
  MODE17/8 -> sum1/32(BFP2)
  MODE17/9 -> sum1/33(BFY2)
  MODE17/10 -> sum1/34(MNL2)
  MODE17/11 -> sum1/35(MNT2)
  MODE17/12 -> sum1/36(MNV2)
  MODE17/13 -> sum1/37(MNR2)
  MODE17/14 -> sum1/38(MNP2)
  MODE17/15 -> sum1/39(MNY2)
  MODE17/16 -> sum1/40(IML2)
  MODE17/17 -> sum1/41(IMT2)
  MODE17/18 -> sum1/42(IMV2)
  MODE17/19 -> sum1/43(IMR2)
  MODE17/20 -> sum1/44(IMP2)
  MODE17/21 -> sum1/45(IMY2)
  MODE17/22 -> sum1/46(TML2)
  MODE17/23 -> sum1/47(TMP2)
  MODE17/24 -> sum1/48(TMY2)
  Demux17/27 -> MODE17/27
  Demux17/28 -> MODE17/28
  Demux17/29 -> MODE17/29
  Demux17/30 -> MODE17/30
  Demux18/1 -> MODE18/1
  Demux18/2 -> MODE18/2
  Demux18/3 -> MODE18/3
  Demux18/4 -> MODE18/4
  Demux18/5 -> MODE18/5
  Demux18/6 -> MODE18/6
  Demux18/7 -> MODE18/7
  Demux18/8 -> MODE18/8
  Demux18/9 -> MODE18/9
  Demux18/10 -> MODE18/10
  Demux18/11 -> MODE18/11
  Demux18/12 -> MODE18/12
  Demux18/13 -> MODE18/13
  Demux18/14 -> MODE18/14
  Demux18/15 -> MODE18/15
  Demux18/16 -> MODE18/16
  Demux18/17 -> MODE18/17
  Demux18/18 -> MODE18/18
  Demux18/19 -> MODE18/19
  Demux18/20 -> MODE18/20
  Demux18/21 -> MODE18/21
  Demux18/22 -> MODE18/22
  Demux18/23 -> MODE18/23
  Demux18/24 -> MODE18/24
  Demux18/25 -> MODE18/25
  Demux18/26 -> MODE18/26
  MODE18/1 -> sum1/49(IPL3)
  MODE18/2 -> sum1/50(IPT3)
  MODE18/3 -> sum1/51(IPY3)
  MODE18/4 -> sum1/52(BFL3)
  MODE18/5 -> sum1/53(BFT3)
  MODE18/6 -> sum1/54(BFV3)
  MODE18/7 -> sum1/55(BFR3)
  MODE18/8 -> sum1/56(BFP3)
  MODE18/9 -> sum1/57(BFY3)
  MODE18/10 -> sum1/58(MNL3)
  MODE18/11 -> sum1/59(MNT3)
  MODE18/12 -> sum1/60(MNV3)
  MODE18/13 -> sum1/61(MNR3)
  MODE18/14 -> sum1/62(MNP3)
  MODE18/15 -> sum1/63(MNY3)
  MODE18/16 -> sum1/64(IML3)
  MODE18/17 -> sum1/65(IMT3)
  MODE18/18 -> sum1/66(IMV3)
  MODE18/19 -> sum1/67(IMR3)
  MODE18/20 -> sum1/68(IMP3)
  MODE18/21 -> sum1/69(IMY3)
  MODE18/22 -> sum1/70(TML3)
  MODE18/23 -> sum1/71(TMP3)
  MODE18/24 -> sum1/72(TMY3)
  Demux18/27 -> MODE18/27
  Demux18/28 -> MODE18/28
  Demux18/29 -> MODE18/29
  Demux18/30 -> MODE18/30
  Demux19/1 -> MODE19/1
  Demux19/2 -> MODE19/2
  Demux19/3 -> MODE19/3
  Demux19/4 -> MODE19/4
  Demux19/5 -> MODE19/5
  Demux19/6 -> MODE19/6
  Demux19/7 -> MODE19/7
  Demux19/8 -> MODE19/8
  Demux19/9 -> MODE19/9
  Demux19/10 -> MODE19/10
  Demux19/11 -> MODE19/11
  Demux19/12 -> MODE19/12
  Demux19/13 -> MODE19/13
  Demux19/14 -> MODE19/14
  Demux19/15 -> MODE19/15
  Demux19/16 -> MODE19/16
  Demux19/17 -> MODE19/17
  Demux19/18 -> MODE19/18
  Demux19/19 -> MODE19/19
  Demux19/20 -> MODE19/20
  Demux19/21 -> MODE19/21
  Demux19/22 -> MODE19/22
  Demux19/23 -> MODE19/23
  Demux19/24 -> MODE19/24
  Demux19/25 -> MODE19/25
  Demux19/26 -> MODE19/26
  MODE19/1 -> sum1/73(IPL4)
  MODE19/2 -> sum1/74(IPT4)
  MODE19/3 -> sum1/75(IPY4)
  MODE19/4 -> sum1/76(BFL4)
  MODE19/5 -> sum1/77(BFT4)
  MODE19/6 -> sum1/78(BFV4)
  MODE19/7 -> sum1/79(BFR4)
  MODE19/8 -> sum1/80(BFP4)
  MODE19/9 -> sum1/81(BFY4)
  MODE19/10 -> sum1/82(MNL4)
  MODE19/11 -> sum1/83(MNT4)
  MODE19/12 -> sum1/84(MNV4)
  MODE19/13 -> sum1/85(MNR4)
  MODE19/14 -> sum1/86(MNP4)
  MODE19/15 -> sum1/87(MNY4)
  MODE19/16 -> sum1/88(IML4)
  MODE19/17 -> sum1/89(IMT4)
  MODE19/18 -> sum1/90(IMV4)
  MODE19/19 -> sum1/91(IMR4)
  MODE19/20 -> sum1/92(IMP4)
  MODE19/21 -> sum1/93(IMY4)
  MODE19/22 -> sum1/94(TML4)
  MODE19/23 -> sum1/95(TMP4)
  MODE19/24 -> sum1/96(TMY4)
  Demux19/27 -> MODE19/27
  Demux19/28 -> MODE19/28
  Demux19/29 -> MODE19/29
  Demux19/30 -> MODE19/30
  MODE20/1 -> sum1/97(IPL5)
  MODE20/2 -> sum1/98(IPT5)
  MODE20/3 -> sum1/99(IPY5)
  MODE20/4 -> sum1/100(BFL5)
  MODE20/5 -> sum1/101(BFT5)
  MODE20/6 -> sum1/102(BFV5)
  MODE20/7 -> sum1/103(BFR5)
  MODE20/8 -> sum1/104(BFP5)
  MODE20/9 -> sum1/105(BFY5)
  MODE20/10 -> sum1/106(MNL5)
  MODE20/11 -> sum1/107(MNT5)
  MODE20/12 -> sum1/108(MNV5)
  MODE20/13 -> sum1/109(MNR5)
  MODE20/14 -> sum1/110(MNP5)
  MODE20/15 -> sum1/111(MNY5)
  MODE20/16 -> sum1/112(IML5)
  MODE20/17 -> sum1/113(IMT5)
  MODE20/18 -> sum1/114(IMV5)
  MODE20/19 -> sum1/115(IMR5)
  MODE20/20 -> sum1/116(IMP5)
  MODE20/21 -> sum1/117(IMY5)
  MODE20/22 -> sum1/118(TML5)
  MODE20/23 -> sum1/119(TMP5)
  MODE20/24 -> sum1/120(TMY5)
  Demux20/1 -> MODE20/1
  Demux20/2 -> MODE20/2
  Demux20/3 -> MODE20/3
  Demux20/4 -> MODE20/4
  Demux20/5 -> MODE20/5
  Demux20/6 -> MODE20/6
  Demux20/7 -> MODE20/7
  Demux20/8 -> MODE20/8
  Demux20/9 -> MODE20/9
  Demux20/10 -> MODE20/10
  Demux20/11 -> MODE20/11
  Demux20/12 -> MODE20/12
  Demux20/13 -> MODE20/13
  Demux20/14 -> MODE20/14
  Demux20/15 -> MODE20/15
  Demux20/16 -> MODE20/16
  Demux20/17 -> MODE20/17
  Demux20/18 -> MODE20/18
  Demux20/19 -> MODE20/19
  Demux20/20 -> MODE20/20
  Demux20/21 -> MODE20/21
  Demux20/22 -> MODE20/22
  Demux20/23 -> MODE20/23
  Demux20/24 -> MODE20/24
  Demux20/25 -> MODE20/25
  Demux20/26 -> MODE20/26
  Demux20/27 -> MODE20/27
  Demux20/28 -> MODE20/28
  Demux20/29 -> MODE20/29
  Demux20/30 -> MODE20/30
  Demux21/1 -> MODE21/1
  Demux21/2 -> MODE21/2
  Demux21/3 -> MODE21/3
  Demux21/4 -> MODE21/4
  Demux21/5 -> MODE21/5
  Demux21/6 -> MODE21/6
  Demux21/7 -> MODE21/7
  Demux21/8 -> MODE21/8
  Demux21/9 -> MODE21/9
  Demux21/10 -> MODE21/10
  Demux21/11 -> MODE21/11
  Demux21/12 -> MODE21/12
  Demux21/13 -> MODE21/13
  Demux21/14 -> MODE21/14
  Demux21/15 -> MODE21/15
  Demux21/16 -> MODE21/16
  Demux21/17 -> MODE21/17
  Demux21/18 -> MODE21/18
  Demux21/19 -> MODE21/19
  Demux21/20 -> MODE21/20
  Demux21/21 -> MODE21/21
  Demux21/22 -> MODE21/22
  Demux21/23 -> MODE21/23
  Demux21/24 -> MODE21/24
  Demux21/25 -> MODE21/25
  Demux21/26 -> MODE21/26
  MODE21/1 -> sum1/121(IPL6)
  MODE21/2 -> sum1/122(IPT6)
  MODE21/3 -> sum1/123(IPY6)
  MODE21/4 -> sum1/124(BFL6)
  MODE21/5 -> sum1/125(BFT6)
  MODE21/6 -> sum1/126(BFV6)
  MODE21/7 -> sum1/127(BFR6)
  MODE21/8 -> sum1/128(BFP6)
  MODE21/9 -> sum1/129(BFY6)
  MODE21/10 -> sum1/130(MNL6)
  MODE21/11 -> sum1/131(MNT6)
  MODE21/12 -> sum1/132(MNV6)
  MODE21/13 -> sum1/133(MNR6)
  MODE21/14 -> sum1/134(MNP6)
  MODE21/15 -> sum1/135(MNY6)
  MODE21/16 -> sum1/136(IML6)
  MODE21/17 -> sum1/137(IMT6)
  MODE21/18 -> sum1/138(IMV6)
  MODE21/19 -> sum1/139(IMR6)
  MODE21/20 -> sum1/140(IMP6)
  MODE21/21 -> sum1/141(IMY6)
  MODE21/22 -> sum1/142(TML6)
  MODE21/23 -> sum1/143(TMP6)
  MODE21/24 -> sum1/144(TMY6)
  Demux21/27 -> MODE21/27
  Demux21/28 -> MODE21/28
  Demux21/29 -> MODE21/29
  Demux21/30 -> MODE21/30
  Demux22/1 -> MODE22/1
  Demux22/2 -> MODE22/2
  Demux22/3 -> MODE22/3
  Demux22/4 -> MODE22/4
  Demux22/5 -> MODE22/5
  Demux22/6 -> MODE22/6
  Demux22/7 -> MODE22/7
  Demux22/8 -> MODE22/8
  Demux22/9 -> MODE22/9
  Demux22/10 -> MODE22/10
  Demux22/11 -> MODE22/11
  Demux22/12 -> MODE22/12
  Demux22/13 -> MODE22/13
  Demux22/14 -> MODE22/14
  Demux22/15 -> MODE22/15
  Demux22/16 -> MODE22/16
  Demux22/17 -> MODE22/17
  Demux22/18 -> MODE22/18
  Demux22/19 -> MODE22/19
  Demux22/20 -> MODE22/20
  Demux22/21 -> MODE22/21
  Demux22/22 -> MODE22/22
  Demux22/23 -> MODE22/23
  Demux22/24 -> MODE22/24
  Demux22/25 -> MODE22/25
  Demux22/26 -> MODE22/26
  MODE22/1 -> sum1/145(IPL7)
  MODE22/2 -> sum1/146(IPT7)
  MODE22/3 -> sum1/147(IPY7)
  MODE22/4 -> sum1/148(BFL7)
  MODE22/5 -> sum1/149(BFT7)
  MODE22/6 -> sum1/150(BFV7)
  MODE22/7 -> sum1/151(BFR7)
  MODE22/8 -> sum1/152(BFP7)
  MODE22/9 -> sum1/153(BFY7)
  MODE22/10 -> sum1/154(MNL7)
  MODE22/11 -> sum1/155(MNT7)
  MODE22/12 -> sum1/156(MNV7)
  MODE22/13 -> sum1/157(MNR7)
  MODE22/14 -> sum1/158(MNP7)
  MODE22/15 -> sum1/159(MNY7)
  MODE22/16 -> sum1/160(IML7)
  MODE22/17 -> sum1/161(IMT7)
  MODE22/18 -> sum1/162(IMV7)
  MODE22/19 -> sum1/163(IMR7)
  MODE22/20 -> sum1/164(IMP7)
  MODE22/21 -> sum1/165(IMY7)
  MODE22/22 -> sum1/166(TML7)
  MODE22/23 -> sum1/167(TMP7)
  MODE22/24 -> sum1/168(TMY7)
  Demux22/27 -> MODE22/27
  Demux22/28 -> MODE22/28
  Demux22/29 -> MODE22/29
  Demux22/30 -> MODE22/30
  Demux23/1 -> MODE23/1
  Demux23/2 -> MODE23/2
  Demux23/3 -> MODE23/3
  Demux23/4 -> MODE23/4
  Demux23/5 -> MODE23/5
  Demux23/6 -> MODE23/6
  Demux23/7 -> MODE23/7
  Demux23/8 -> MODE23/8
  Demux23/9 -> MODE23/9
  Demux23/10 -> MODE23/10
  Demux23/11 -> MODE23/11
  Demux23/12 -> MODE23/12
  Demux23/13 -> MODE23/13
  Demux23/14 -> MODE23/14
  Demux23/15 -> MODE23/15
  Demux23/16 -> MODE23/16
  Demux23/17 -> MODE23/17
  Demux23/18 -> MODE23/18
  Demux23/19 -> MODE23/19
  Demux23/20 -> MODE23/20
  Demux23/21 -> MODE23/21
  Demux23/22 -> MODE23/22
  Demux23/23 -> MODE23/23
  Demux23/24 -> MODE23/24
  Demux23/25 -> MODE23/25
  Demux23/26 -> MODE23/26
  MODE23/1 -> sum1/169(IPL8)
  MODE23/2 -> sum1/170(IPT8)
  MODE23/3 -> sum1/171(IPY8)
  MODE23/4 -> sum1/172(BFL8)
  MODE23/5 -> sum1/173(BFT8)
  MODE23/6 -> sum1/174(BFV8)
  MODE23/7 -> sum1/175(BFR8)
  MODE23/8 -> sum1/176(BFP8)
  MODE23/9 -> sum1/177(BFY8)
  MODE23/10 -> sum1/178(MNL8)
  MODE23/11 -> sum1/179(MNT8)
  MODE23/12 -> sum1/180(MNV8)
  MODE23/13 -> sum1/181(MNR8)
  MODE23/14 -> sum1/182(MNP8)
  MODE23/15 -> sum1/183(MNY8)
  MODE23/16 -> sum1/184(IML8)
  MODE23/17 -> sum1/185(IMT8)
  MODE23/18 -> sum1/186(IMV8)
  MODE23/19 -> sum1/187(IMR8)
  MODE23/20 -> sum1/188(IMP8)
  MODE23/21 -> sum1/189(IMY8)
  MODE23/22 -> sum1/190(TML8)
  MODE23/23 -> sum1/191(TMP8)
  MODE23/24 -> sum1/192(TMY8)
  Demux23/27 -> MODE23/27
  Demux23/28 -> MODE23/28
  Demux23/29 -> MODE23/29
  Demux23/30 -> MODE23/30
  MODE24/10 -> sum1/202(MNL9)
  MODE24/11 -> sum1/203(MNT9)
  MODE24/12 -> sum1/204(MNV9)
  MODE24/13 -> sum1/205(MNR9)
  MODE24/14 -> sum1/206(MNP9)
  MODE24/15 -> sum1/207(MNY9)
  MODE24/16 -> sum1/208(IML9)
  MODE24/17 -> sum1/209(IMT9)
  MODE24/18 -> sum1/210(IMV9)
  MODE24/19 -> sum1/211(IMR9)
  MODE24/20 -> sum1/212(IMP9)
  MODE24/21 -> sum1/213(IMY9)
  MODE24/22 -> sum1/214(TML9)
  MODE24/23 -> sum1/215(TMP9)
  MODE24/24 -> sum1/216(TMY9)
  Demux24/11 -> MODE24/11
  Demux24/12 -> MODE24/12
  Demux24/13 -> MODE24/13
  Demux24/14 -> MODE24/14
  Demux24/15 -> MODE24/15
  Demux24/16 -> MODE24/16
  Demux24/17 -> MODE24/17
  Demux24/18 -> MODE24/18
  Demux24/19 -> MODE24/19
  Demux24/20 -> MODE24/20
  Demux24/21 -> MODE24/21
  Demux24/22 -> MODE24/22
  Demux24/23 -> MODE24/23
  Demux24/24 -> MODE24/24
  Demux24/25 -> MODE24/25
  Demux24/26 -> MODE24/26
  Demux24/27 -> MODE24/27
  Demux24/28 -> MODE24/28
  Demux24/29 -> MODE24/29
  Demux24/30 -> MODE24/30
  Demux14/1 -> MODE14/1
  Demux14/2 -> MODE14/2
  Demux14/3 -> MODE14/3
  Demux14/4 -> MODE14/4
  Demux14/5 -> MODE14/5
  Demux14/6 -> MODE14/6
  Demux14/7 -> MODE14/7
  Demux14/8 -> MODE14/8
  Demux14/9 -> MODE14/9
  Demux14/10 -> MODE14/10
  Demux14/11 -> MODE14/11
  Demux14/12 -> MODE14/12
  Demux14/13 -> MODE14/13
  Demux14/14 -> MODE14/14
  Demux14/15 -> MODE14/15
  Demux14/16 -> MODE14/16
  Demux14/17 -> MODE14/17
  Demux14/18 -> MODE14/18
  Demux14/19 -> MODE14/19
  Demux14/20 -> MODE14/20
  Demux14/21 -> MODE14/21
  Demux14/22 -> MODE14/22
  Demux14/23 -> MODE14/23
  Demux14/24 -> MODE14/24
  Demux14/25 -> MODE14/25
  Demux14/26 -> MODE14/26
  MODE14/1 -> sum1/217(IPL10)
  MODE14/2 -> sum1/218(IPT10)
  MODE14/3 -> sum1/219(IPY10)
  MODE14/4 -> sum1/220(BFL10)
  MODE14/5 -> sum1/221(BFT10)
  MODE14/6 -> sum1/222(BFV10)
  MODE14/7 -> sum1/223(BFR10)
  MODE14/8 -> sum1/224(BFP10)
  MODE14/9 -> sum1/225(BFY10)
  MODE14/10 -> sum1/226(MNL10)
  MODE14/11 -> sum1/227(MNT10)
  MODE14/12 -> sum1/228(MNV10)
  MODE14/13 -> sum1/229(MNR10)
  MODE14/14 -> sum1/230(MNP10)
  MODE14/15 -> sum1/231(MNY10)
  MODE14/16 -> sum1/232(IML10)
  MODE14/17 -> sum1/233(IMT10)
  MODE14/18 -> sum1/234(IMV10)
  MODE14/19 -> sum1/235(IMR10)
  MODE14/20 -> sum1/236(IMP10)
  MODE14/21 -> sum1/237(IMY10)
  MODE14/22 -> sum1/238(TML10)
  MODE14/23 -> sum1/239(TMP10)
  MODE14/24 -> sum1/240(TMY10)
  Demux14/27 -> MODE14/27
  Demux14/28 -> MODE14/28
  Demux14/29 -> MODE14/29
  Demux14/30 -> MODE14/30
  Demux15/1 -> MODE15/1
  Demux15/2 -> MODE15/2
  Demux15/3 -> MODE15/3
  Demux15/4 -> MODE15/4
  Demux15/5 -> MODE15/5
  Demux15/6 -> MODE15/6
  Demux15/7 -> MODE15/7
  Demux15/8 -> MODE15/8
  Demux15/9 -> MODE15/9
  Demux15/10 -> MODE15/10
  Demux15/11 -> MODE15/11
  Demux15/12 -> MODE15/12
  Demux15/13 -> MODE15/13
  Demux15/14 -> MODE15/14
  Demux15/15 -> MODE15/15
  Demux15/16 -> MODE15/16
  Demux15/17 -> MODE15/17
  Demux15/18 -> MODE15/18
  Demux15/19 -> MODE15/19
  Demux15/20 -> MODE15/20
  Demux15/21 -> MODE15/21
  Demux15/22 -> MODE15/22
  Demux15/23 -> MODE15/23
  Demux15/24 -> MODE15/24
  Demux15/25 -> MODE15/25
  Demux15/26 -> MODE15/26
  MODE15/1 -> sum1/241(IPL11)
  MODE15/2 -> sum1/242(IPT11)
  MODE15/3 -> sum1/243(IPY11)
  MODE15/4 -> sum1/244(BFL11)
  MODE15/5 -> sum1/245(BFT11)
  MODE15/6 -> sum1/246(BFV11)
  MODE15/7 -> sum1/247(BFR11)
  MODE15/8 -> sum1/248(BFP11)
  MODE15/9 -> sum1/249(BFY11)
  MODE15/10 -> sum1/250(MNL11)
  MODE15/11 -> sum1/251(MNT11)
  MODE15/12 -> sum1/252(MNV11)
  MODE15/13 -> sum1/253(MNR11)
  MODE15/14 -> sum1/254(MNP11)
  MODE15/15 -> sum1/255(MNY11)
  MODE15/16 -> sum1/256(IML11)
  MODE15/17 -> sum1/257(IMT11)
  MODE15/18 -> sum1/258(IMV11)
  MODE15/19 -> sum1/259(IMR11)
  MODE15/20 -> sum1/260(IMP11)
  MODE15/21 -> sum1/261(IMY11)
  MODE15/22 -> sum1/262(TML11)
  MODE15/23 -> sum1/263(TMP11)
  MODE15/24 -> sum1/264(TMY11)
  Demux15/27 -> MODE15/27
  Demux15/28 -> MODE15/28
  Demux15/29 -> MODE15/29
  Demux15/30 -> MODE15/30
  Demux16/1 -> MODE16/1
  Demux16/2 -> MODE16/2
  Demux16/3 -> MODE16/3
  Demux16/4 -> MODE16/4
  Demux16/5 -> MODE16/5
  Demux16/6 -> MODE16/6
  Demux16/7 -> MODE16/7
  Demux16/8 -> MODE16/8
  Demux16/9 -> MODE16/9
  Demux16/10 -> MODE16/10
  Demux16/11 -> MODE16/11
  Demux16/12 -> MODE16/12
  Demux16/13 -> MODE16/13
  Demux16/14 -> MODE16/14
  Demux16/15 -> MODE16/15
  Demux16/16 -> MODE16/16
  Demux16/17 -> MODE16/17
  Demux16/18 -> MODE16/18
  Demux16/19 -> MODE16/19
  Demux16/20 -> MODE16/20
  Demux16/21 -> MODE16/21
  Demux16/22 -> MODE16/22
  Demux16/23 -> MODE16/23
  Demux16/24 -> MODE16/24
  Demux16/25 -> MODE16/25
  Demux16/26 -> MODE16/26
  MODE16/1 -> sum1/265(IPL12)
  MODE16/2 -> sum1/266(IPT12)
  MODE16/3 -> sum1/267(IPY12)
  MODE16/4 -> sum1/268(BFL12)
  MODE16/5 -> sum1/269(BFT12)
  MODE16/6 -> sum1/270(BFV12)
  MODE16/7 -> sum1/271(BFR12)
  MODE16/8 -> sum1/272(BFP12)
  MODE16/9 -> sum1/273(BFY12)
  MODE16/10 -> sum1/274(MNL12)
  MODE16/11 -> sum1/275(MNT12)
  MODE16/12 -> sum1/276(MNV12)
  MODE16/13 -> sum1/277(MNR12)
  MODE16/14 -> sum1/278(MNP12)
  MODE16/15 -> sum1/279(MNY12)
  MODE16/16 -> sum1/280(IML12)
  MODE16/17 -> sum1/281(IMT12)
  MODE16/18 -> sum1/282(IMV12)
  MODE16/19 -> sum1/283(IMR12)
  MODE16/20 -> sum1/284(IMP12)
  MODE16/21 -> sum1/285(IMY12)
  MODE16/22 -> sum1/286(TML12)
  MODE16/23 -> sum1/287(TMP12)
  MODE16/24 -> sum1/288(TMY12)
  Demux16/27 -> MODE16/27
  Demux16/28 -> MODE16/28
  Demux16/29 -> MODE16/29
  Demux16/30 -> MODE16/30
  [Signal] -> Demux13/1, Demux17/1, Demux18/1, Demux19/1, Demux20/1, Demux21/1, Demux22/1, Demux24/1, Demux14/1, Demux15/1, Demux16/1, Demux23/1
  MODE24/1 -> sum1/193(IPL9)
  MODE24/2 -> sum1/194(IPT9)
  MODE24/3 -> sum1/195(IPY9)
  MODE24/4 -> sum1/196(BFL9)
  MODE24/5 -> sum1/197(BFT9)
  MODE24/6 -> sum1/198(BFV9)
  MODE24/7 -> sum1/199(BFR9)
  MODE24/8 -> sum1/200(BFP9)
  MODE24/9 -> sum1/201(BFY9)
  Demux24/1 -> MODE24/1
  Demux24/2 -> MODE24/2
  Demux24/3 -> MODE24/3
  Demux24/4 -> MODE24/4
  Demux24/5 -> MODE24/5
  Demux24/6 -> MODE24/6
  Demux24/7 -> MODE24/7
  Demux24/8 -> MODE24/8
  Demux24/9 -> MODE24/9
  Demux24/10 -> MODE24/10
  [Signal] -> Demux2/1, Demux3/1, Demux4/1, Demux5/1, Demux6/1, Demux7/1, Demux8/1, Demux9/1, Demux10/1, Demux11/1, Demux12/1, Demux/1
  Mux1/1 -> [SUM1]
  Mux2/1 -> [SUM2]
  [SUM1] -> Demux1/1
  [SUM2] -> Demux25/1
  Demux1/1 -> sum2/1(IPL1)
  Demux1/2 -> sum2/2(IPT1)
  Demux1/3 -> sum2/3(IPY1)
  Demux1/4 -> sum2/4(BFL1)
  Demux1/5 -> sum2/5(BFT1)
  Demux1/6 -> sum2/6(BFV1)
  Demux1/7 -> sum2/7(BFR1)
  Demux1/8 -> sum2/8(BFP1)
  Demux1/9 -> sum2/9(BFY1)
  Demux1/10 -> sum2/10(MNL1)
  Demux1/11 -> sum2/11(MNT1)
  Demux1/12 -> sum2/12(MNV1)
  Demux1/13 -> sum2/13(MNR1)
  Demux1/14 -> sum2/14(MNP1)
  Demux1/15 -> sum2/15(MNY1)
  Demux1/16 -> sum2/16(IML1)
  Demux1/17 -> sum2/17(IMT1)
  Demux1/18 -> sum2/18(IMV1)
  Demux1/19 -> sum2/19(IMR1)
  Demux1/20 -> sum2/20(IMP1)
  Demux1/21 -> sum2/21(IMY1)
  Demux1/22 -> sum2/22(TML1)
  Demux1/23 -> sum2/23(TMP1)
  Demux1/24 -> sum2/24(TMY1)
  Demux25/1 -> sum2/25(IPL2)
  Demux25/2 -> sum2/26(IPT2)
  Demux25/3 -> sum2/27(IPY2)
  Demux25/4 -> sum2/28(BFL2)
  Demux25/5 -> sum2/29(BFT2)
  Demux25/6 -> sum2/30(BFV2)
  Demux25/7 -> sum2/31(BFR2)
  Demux25/8 -> sum2/32(BFP2)
  Demux25/9 -> sum2/33(BFY2)
  Demux25/10 -> sum2/34(MNL2)
  Demux25/11 -> sum2/35(MNT2)
  Demux25/12 -> sum2/36(MNV2)
  Demux25/17 -> sum2/41(IMT2)
  Demux25/18 -> sum2/42(IMV2)
  Demux25/19 -> sum2/43(IMR2)
  Demux25/20 -> sum2/44(IMP2)
  sum2/1(IPL) -> Mux5/1
  sum2/2(IPT) -> Mux5/2
  sum2/3(IPY) -> Mux5/3
  sum2/4(BFL) -> Mux5/4
  sum2/5(BFT) -> Mux5/5
  sum2/6(BFV) -> Mux5/6
  sum2/7(BFR) -> Mux5/7
  sum2/8(BFP) -> Mux5/8
  sum2/9(BFY) -> Mux5/9
  sum2/10(MNL) -> Mux5/10
  sum2/11(MNT) -> Mux5/11
  sum2/12(MNV) -> Mux5/12
  sum2/13(MNR) -> Mux5/13
  sum2/14(MNP) -> Mux5/14
  sum2/15(MNY) -> Mux5/15
  sum2/16(IML) -> Mux5/16
  sum2/17(IMT) -> Mux5/17
  sum2/18(IMV) -> Mux5/18
  sum2/19(IMR) -> Mux5/19
  sum2/20(IMP) -> Mux5/20
  sum2/21(IMY) -> Mux5/21
  sum2/22(TML) -> Mux5/22
  sum2/23(TMP) -> Mux5/23
  sum2/24(TMY) -> Mux5/24
  Demux25/13 -> sum2/37(MNR2)
  Demux25/14 -> sum2/38(MNP2)
  Demux25/15 -> sum2/39(MNY2)
  Demux25/16 -> sum2/40(IML2)
  Demux25/21 -> sum2/45(IMY2)
  Demux25/22 -> sum2/46(TML2)
  Demux25/23 -> sum2/47(TMP2)
  Demux25/24 -> sum2/48(TMY2)
  Mux5/1 -> Demux26/1
  Demux26/1 -> sum10/1(IPL1)
  Demux26/2 -> sum10/2(IPT1)
  Demux26/3 -> sum10/3(IPY1)
  Demux26/4 -> sum10/4(BFL1)
  Demux26/5 -> sum10/5(BFT1)
  Demux26/6 -> sum10/6(BFV1)
  Demux26/7 -> sum10/7(BFR1)
  Demux26/8 -> sum10/8(BFP1)
  Demux26/9 -> sum10/9(BFY1)
  Demux26/10 -> sum10/10(MNL1)
  Demux26/11 -> sum10/11(MNT1)
  Demux26/12 -> sum10/12(MNV1)
  Demux26/13 -> sum10/13(MNR1)
  Demux26/14 -> sum10/14(MNP1)
  Demux26/15 -> sum10/15(MNY1)
  Demux26/16 -> sum10/16(IML1)
  Demux26/17 -> sum10/17(IMT1)
  Demux26/18 -> sum10/18(IMV1)
  Demux26/19 -> sum10/19(IMR1)
  Demux26/20 -> sum10/20(IMP1)
  Demux26/21 -> sum10/21(IMY1)
  Demux26/22 -> sum10/22(TML1)
  Demux26/23 -> sum10/23(TMP1)
  Demux26/24 -> sum10/24(TMY1)
  IPDC/1(LEN_OUT) -> sum10/49(IPL3)
  IPDC/2(PIT_OUT) -> sum10/50(IPT3)
  IPDC/3(YAW_OUT) -> sum10/51(IPY3)
  F0/1 -> DIAG/34
  F1/1 -> DIAG/35
  F2/1 -> DIAG/36
  F3/1 -> DIAG/37
  BF/1 -> DIAG/38
  Demux28/1 -> GAS_MODE1/1
  Demux28/2 -> GAS_MODE1/2
  Demux28/3 -> GAS_MODE1/3
  Demux28/4 -> GAS_MODE1/4
  Demux28/5 -> GAS_MODE1/5
  Demux28/6 -> GAS_MODE1/6
  Demux30/5 -> GAS_MODE2/5
  Demux30/6 -> GAS_MODE2/6
  Demux31/5 -> GAS_MODE3/5
  Demux31/6 -> GAS_MODE3/6
  Demux32/5 -> GAS_MODE4/5
  Demux32/6 -> GAS_MODE4/6
  Demux33/5 -> GAS_MODE5/5
  Demux33/6 -> GAS_MODE5/6
  Demux30/1 -> GAS_MODE2/1
  Demux30/2 -> GAS_MODE2/2
  Demux30/3 -> GAS_MODE2/3
  Demux30/4 -> GAS_MODE2/4
  Demux30/7 -> GAS_MODE2/7
  Demux31/1 -> GAS_MODE3/1
  Demux31/2 -> GAS_MODE3/2
  Demux31/3 -> GAS_MODE3/3
  Demux31/4 -> GAS_MODE3/4
  Demux31/7 -> GAS_MODE3/7
  Demux32/1 -> GAS_MODE4/1
  Demux32/2 -> GAS_MODE4/2
  Demux32/3 -> GAS_MODE4/3
  Demux32/4 -> GAS_MODE4/4
  Demux32/7 -> GAS_MODE4/7
  Demux33/1 -> GAS_MODE5/1
  Demux33/2 -> GAS_MODE5/2
  Demux33/3 -> GAS_MODE5/3
  Demux33/4 -> GAS_MODE5/4
  Demux33/7 -> GAS_MODE5/7
  Demux28/7 -> GAS_MODE1/7
  GAS_MODE1/1 -> Subsystem/1(M1_1)
  GAS_MODE1/2 -> Subsystem/2(M2_1)
  GAS_MODE1/3 -> Subsystem/3(M3_1)
  GAS_MODE1/4 -> Subsystem/4(M4_1)
  GAS_MODE1/5 -> Subsystem/5(M5_1)
  GAS_MODE2/1 -> Subsystem/6(M1_2)
  GAS_MODE2/2 -> Subsystem/7(M2_2)
  GAS_MODE2/3 -> Subsystem/8(M3_2)
  GAS_MODE2/4 -> Subsystem/9(M4_2)
  GAS_MODE2/5 -> Subsystem/10(M5_2)
  GAS_MODE3/1 -> Subsystem/11(M1_3)
  GAS_MODE3/2 -> Subsystem/12(M2_3)
  GAS_MODE3/3 -> Subsystem/13(M3_3)
  GAS_MODE3/4 -> Subsystem/14(M4_3)
  GAS_MODE3/5 -> Subsystem/15(M5_3)
  GAS_MODE4/1 -> Subsystem/16(M1_4)
  GAS_MODE4/2 -> Subsystem/17(M2_4)
  GAS_MODE4/3 -> Subsystem/18(M3_4)
  GAS_MODE4/4 -> Subsystem/19(M4_4)
  GAS_MODE4/5 -> Subsystem/20(M5_4)
  GAS_MODE5/1 -> Subsystem/21(M1_5)
  GAS_MODE5/2 -> Subsystem/22(M2_5)
  GAS_MODE5/3 -> Subsystem/23(M3_5)
  GAS_MODE5/4 -> Subsystem/24(M4_5)
  GAS_MODE5/5 -> Subsystem/25(M5_5)
  DIAG/35 -> Mux3/5
  DIAG/34 -> Mux3/4
  DIAG/33 -> Mux3/3
  DIAG/32 -> Mux3/2
  DIAG/31 -> Mux3/1
  Mux3/1 -> [Signal_GAS_M]
  Mux6/1 -> DRIVEDECPL_GAS/1
  DRIVEDECPL_GAS/1 -> Demux34/1
  Mux11/1 -> EUL2COIL_GAS/1
  EUL2COIL_GAS/1 -> Demux35/1
  Demux34/2 -> Mux11/2
  Demux34/3 -> Mux11/3
  Demux34/4 -> Mux11/4
  Demux34/5 -> Mux11/5
  Demux34/1 -> Mux11/1
  SUM_GAS/1(M1_OUT) -> Mux6/1
  SUM_GAS/2(M2_OUT) -> Mux6/2
  SUM_GAS/3(M3_OUT) -> Mux6/3
  SUM_GAS/4(M4_OUT) -> Mux6/4
  SUM_GAS/5(M5_OUT) -> Mux6/5
  Subsystem/1(Out1) -> Mux7/1
  Subsystem/2(Out2) -> Mux7/2
  Subsystem/3(Out3) -> Mux7/3
  Subsystem/4(Out4) -> Mux7/4
  Subsystem/5(Out5) -> Mux7/5
  Mux7/1 -> Demux36/1
  Demux36/1 -> AI_GAS/1(M1_IN)
  Demux36/2 -> AI_GAS/2(M2_IN)
  Demux36/3 -> AI_GAS/3(M3_IN)
  Demux36/4 -> AI_GAS/4(M4_IN)
  Demux36/5 -> AI_GAS/5(M5_IN)
  AI_GAS/1(M1_OUT) -> SUM_GAS/1(M1_IN)
  AI_GAS/2(M2_OUT) -> SUM_GAS/2(M2_IN)
  AI_GAS/3(M3_OUT) -> SUM_GAS/3(M3_IN)
  AI_GAS/4(M4_OUT) -> SUM_GAS/4(M4_IN)
  AI_GAS/5(M5_OUT) -> SUM_GAS/5(M5_IN)
  sum10/1(IPL) -> Mux9/1
  sum10/2(IPT) -> Mux9/2
  sum10/3(IPY) -> Mux9/3
  sum10/4(BFL) -> Mux9/4
  sum10/5(BFT) -> Mux9/5
  sum10/6(BFV) -> Mux9/6
  sum10/7(BFR) -> Mux9/7
  sum10/8(BFP) -> Mux9/8
  sum10/9(BFY) -> Mux9/9
  sum10/10(MNL) -> Mux9/10
  sum10/11(MNT) -> Mux9/11
  sum10/12(MNV) -> Mux9/12
  sum10/13(MNR) -> Mux9/13
  sum10/14(MNP) -> Mux9/14
  sum10/15(MNY) -> Mux9/15
  sum10/16(IML) -> Mux9/16
  sum10/17(IMT) -> Mux9/17
  sum10/18(IMV) -> Mux9/18
  sum10/19(IMR) -> Mux9/19
  sum10/20(IMP) -> Mux9/20
  sum10/21(IMY) -> Mux9/21
  sum10/22(TML) -> Mux9/22
  sum10/23(TMP) -> Mux9/23
  sum10/24(TMY) -> Mux9/24
  Mux10/1 -> QUAEXC_SEL/1
  QUAEXC_SEL/1 -> Demux40/1
  Demux39/1 -> sum3/1(IPL1)
  Demux39/2 -> sum3/2(IPT1)
  Demux39/3 -> sum3/3(IPY1)
  Demux39/4 -> sum3/4(BFL1)
  Demux39/5 -> sum3/5(BFT1)
  Demux39/6 -> sum3/6(BFV1)
  Demux39/7 -> sum3/7(BFR1)
  Demux39/8 -> sum3/8(BFP1)
  Demux39/9 -> sum3/9(BFY1)
  Demux39/10 -> sum3/10(MNL1)
  Demux39/11 -> sum3/11(MNT1)
  Demux39/12 -> sum3/12(MNV1)
  Demux39/13 -> sum3/13(MNR1)
  Demux39/14 -> sum3/14(MNP1)
  Demux39/15 -> sum3/15(MNY1)
  Demux39/16 -> sum3/16(IML1)
  Demux39/17 -> sum3/17(IMT1)
  Demux39/18 -> sum3/18(IMV1)
  Demux39/19 -> sum3/19(IMR1)
  Demux39/20 -> sum3/20(IMP1)
  Demux39/21 -> sum3/21(IMY1)
  Demux39/22 -> sum3/22(TML1)
  Demux39/23 -> sum3/23(TMP1)
  Demux39/24 -> sum3/24(TMY1)
  Demux40/2 -> sum3/26(IPT2)
  Demux40/3 -> sum3/27(IPY2)
  Demux40/4 -> sum3/28(BFL2)
  Demux40/5 -> sum3/29(BFT2)
  Demux40/6 -> sum3/30(BFV2)
  Demux40/7 -> sum3/31(BFR2)
  Demux40/8 -> sum3/32(BFP2)
  Demux40/9 -> sum3/33(BFY2)
  Demux40/10 -> sum3/34(MNL2)
  Demux40/11 -> sum3/35(MNT2)
  Demux40/12 -> sum3/36(MNV2)
  Demux40/13 -> sum3/37(MNR2)
  Demux40/14 -> sum3/38(MNP2)
  Demux40/15 -> sum3/39(MNY2)
  Demux40/16 -> sum3/40(IML2)
  Demux40/17 -> sum3/41(IMT2)
  Demux40/18 -> sum3/42(IMV2)
  Demux40/19 -> sum3/43(IMR2)
  Demux40/20 -> sum3/44(IMP2)
  Demux40/21 -> sum3/45(IMY2)
  Demux40/22 -> sum3/46(TML2)
  Demux40/23 -> sum3/47(TMP2)
  Demux40/24 -> sum3/48(TMY2)
  Demux40/1 -> sum3/25(IPL2)
  Mux9/1 -> Demux39/1
  QUAEXC/1 -> Mux10/1
  Ground8/1 -> sum3/49(BFL3)
  Ground9/1 -> sum3/50(BFP3)
  Ground11/1 -> sum3/51(BFY3)
  Ground13/1 -> sum3/55(IPL3)
  Ground15/1 -> sum3/56(IPT3)
  Ground18/1 -> sum3/57(IPY3)
  sum3/24(TMY) -> TMYo/1
  sum3/1(IPL) -> IPLo/1
  sum3/2(IPT) -> IPTo/1
  sum3/3(IPY) -> IPYo/1
  sum3/4(BFL) -> BFLo/1
  sum3/5(BFT) -> BFTo/1
  sum3/6(BFV) -> BFVo/1
  sum3/7(BFR) -> BFRo/1
  sum3/8(BFP) -> BFPo/1
  sum3/9(BFY) -> BFYo/1
  sum3/10(MNL) -> MNLo/1
  sum3/11(MNT) -> MNTo/1
  sum3/12(MNV) -> MNVo/1
  sum3/13(MNR) -> MNRo/1
  sum3/14(MNP) -> MNPo/1
  sum3/15(MNY) -> MNYo/1
  sum3/16(IML) -> IMLo/1
  sum3/17(IMT) -> IMTo/1
  sum3/18(IMV) -> IMVo/1
  sum3/19(IMR) -> IMRo/1
  sum3/20(IMP) -> IMPo/1
  sum3/21(IMY) -> IMYo/1
  sum3/22(TML) -> TMLo/1
  sum3/23(TMP) -> TMPo/1
  Demux40/25 -> Mux13/1
  Demux40/26 -> Mux13/2
  Demux40/27 -> Mux13/3
  Demux40/28 -> Mux13/4
  Demux40/29 -> Mux13/5
  Demux38/1 -> Subsystem/26(M1_6)
  Demux38/2 -> Subsystem/27(M2_6)
  Demux38/3 -> Subsystem/28(M3_6)
  Demux38/4 -> Subsystem/29(M4_6)
  Demux38/5 -> Subsystem/30(M5_6)
  Mux13/1 -> [GASEXC]
  [GASEXC] -> Demux38/1
  Demux41/1 -> DAMP_GAS/1
  Demux41/2 -> DAMP_GAS/2
  Demux41/3 -> DAMP_GAS/3
  Demux41/4 -> DAMP_GAS/4
  Demux41/5 -> DAMP_GAS/5
  [Signal_GAS_M] -> Demux41/1, Demux33/1, Demux32/1, Demux31/1, Demux30/1, Demux28/1
  Demux41/6 -> Terminator/1
  Demux41/7 -> ?
  DAMP_GAS/5 -> Subsystem/35(M5_7)
  DAMP_GAS/1 -> Subsystem/31(M1_7)
  DAMP_GAS/4 -> Subsystem/34(M4_7)
  DAMP_GAS/3 -> Subsystem/33(M3_7)
  DAMP_GAS/2 -> Subsystem/32(M2_7)
  GASDC/1(M1_OUT) -> Sum5/2
  GASDC/2(M2_OUT) -> Sum6/2
  GASDC/3(M3_OUT) -> Sum7/2
  GASDC/4(M4_OUT) -> Sum8/2
  GASDC/5(M5_OUT) -> Sum9/2
  Demux37/1 -> GASDC/1(F0_IN)
  Demux37/2 -> GASDC/2(F1_IN)
  Demux37/3 -> GASDC/3(F2_IN)
  Demux37/4 -> GASDC/4(F3_IN)
  Demux37/5 -> GASDC/5(BF_IN)
  [GASDC] -> Demux37/1
  DIAG/36 -> Mux8/1
  DIAG/37 -> Mux8/2
  DIAG/38 -> Mux8/3
  DIAG/39 -> Mux8/4
  DIAG/40 -> Mux8/5
  Mux8/1 -> [GASDC]
  Demux35/1 -> Sum5/1
  Demux35/2 -> Sum6/1
  Demux35/3 -> Sum7/1
  Demux35/4 -> Sum8/1
  Demux35/5 -> Sum9/1
  COILOUT_GAS/1(F0_OUT) -> F0out/1
  COILOUT_GAS/2(F1_OUT) -> F1out/1
  COILOUT_GAS/3(F2_OUT) -> F2out/1
  COILOUT_GAS/4(F3_OUT) -> F3out/1
  COILOUT_GAS/5(BF_OUT) -> BFout/1
  Sum9/1 -> COILOUT_GAS/5(BF_IN)
  Sum8/1 -> COILOUT_GAS/4(F3_IN)
  Sum7/1 -> COILOUT_GAS/3(F2_IN)
  Sum6/1 -> COILOUT_GAS/2(F1_IN)
  Sum5/1 -> COILOUT_GAS/1(F0_IN)
  TMOL/1(BFL) -> sum10/52(BFL3)
  TMOL/2(BFP) -> sum10/53(BFP3)
  TMOL/3(BFY) -> sum10/54(BFY3)
  TMOL/4(MNL) -> sum10/55(MNL3)
  TMOL/5(MNP) -> sum10/56(MNP3)
  TMOL/6(MNY) -> sum10/57(MNY3)
  TMOL/7(IML) -> sum10/58(IML3)
  TMOL/8(IMP) -> sum10/59(IMP3)
  TMOL/9(IMY) -> sum10/60(IMY3)
  TMOL/10(TML) -> sum10/61(TML3)
  TMOL/11(TMP) -> sum10/62(TMP3)
  TMOL/12(TMY) -> sum10/63(TMY3)
  Demux27/25 -> TMOL/1(OLL), DAMP/25(TML)
  Mux12/1 -> [Signal_MNOL]
  DIAG/41 -> Mux12/1
  DIAG/42 -> Mux12/2
  DIAG/43 -> Mux12/3
  DIAG/44 -> Mux12/4
  DIAG/45 -> Mux12/5
  DIAG/46 -> Mux12/6
  [Signal_MNOL] -> Demux42/1
  Demux42/2 -> Terminator1/1
  Demux42/3 -> Terminator2/1
  Demux42/4 -> Terminator3/1
  Demux42/1 -> MNOL_SERVO_MN/1(LEN_IN)
  Demux42/5 -> MNOL_SERVO_MN/2(PIT_IN)
  Demux42/6 -> MNOL_SERVO_MN/3(YAW_IN)
  MNOL_SERVO_MN/1(LEN_OUT) -> sum3/52(MNL3)
  MNOL_SERVO_MN/2(PIT_OUT) -> sum3/53(MNP3)
  MNOL_SERVO_MN/3(YAW_OUT) -> sum3/54(MNY3)
